simulink model "Lab8a"  (Simulink 7.4)
settings: Solver=ode23tb  StartTime=0.0  StopTime=0.2  MaxStep=100e-6  RelTol=1e-3
libraries: powerlib x5, powerlib_extras x2
settings Model: Creator=msse9  LastModifiedBy=msse9

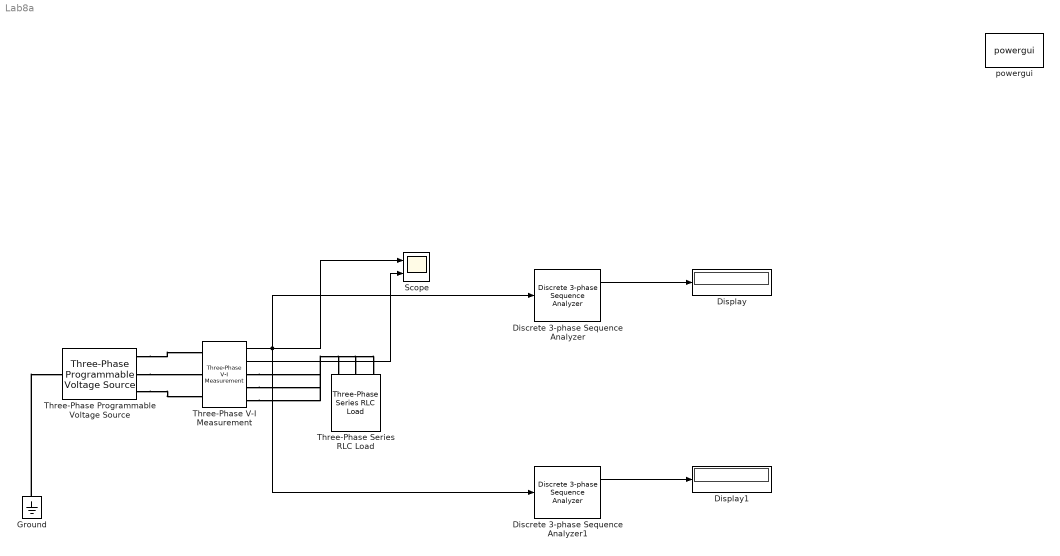
== system Lab8a ==
  Discrete 3-phase Sequence Analyzer : powerlib_extras/Discrete Measurements/Discrete 3-phase Sequence Analyzer  DialogController=POWERSYS.PowerSysDialog  SystemSampleTime=-1  Freq=50  n=3  seq=Zero  Par_Init=[0 0]  Ts=50e-6
  Discrete 3-phase Sequence Analyzer1 : powerlib_extras/Discrete Measurements/Discrete 3-phase Sequence Analyzer  DialogController=POWERSYS.PowerSysDialog  SystemSampleTime=-1  Freq=50  n=1  seq=Positive  Par_Init=[0 0]  Ts=50e-6
  Display : Display
  Display1 : Display
  Ground : powerlib/Elements/Ground  DialogController=POWERSYS.PowerSysDialog  PhysicalDomain=powersysdomain  SubClassName=unknown  LeftPortType=p1  RightPortType=p1  LConnTagsString=a
  Scope : Scope  NumInputPorts=2
      settings: YMin=-5~-5  YMax=5~5  SaveName=Lab8  SampleInput=on  SampleTime=100e-6
  Three-Phase Programmable Voltage Source : powerlib/Electrical Sources/Three-Phase Programmable Voltage Source  DialogController=POWERSYS.PowerSysDialog  SystemSampleTime=-1  PositiveSequence="[400  0 50]"  VariationEntity=None  VariationType=Step  VariationStep=0.5  VariationRate=10  VariationMagnitude=0.3  VariationFrequency=2  VariationTiming=[1 2]  VariationPhaseA=off  Amplitudes=[1 0.8 1.2 1.0]  TimeValues=[0 0.1 0.15 0.2]  HarmonicGeneration=on  HarmonicA=[3 0.2 0 0]  HarmonicB=[5 0.3 0 2]  Timing="[0.1  1]"
  Three-Phase Series RLC Load : powerlib/Elements/Three-Phase Series RLC Load  DialogController=POWERSYS.PowerSysDialog  PhysicalDomain=powersysdomain  SubClassName=unknown  LeftPortType=p1  RightPortType=p1  LConnTagsString=A|B|C  Configuration=Y (grounded)  NominalVoltage=400  NominalFrequency=50  ActivePower=1000  InductivePower=1000  CapacitivePower=0  Measurements=None
  Three-Phase V-I Measurement : powerlib/Measurements/Three-Phase V-I Measurement  DialogController=POWERSYS.PowerSysDialog  SystemSampleTime=-1  VoltageMeasurement=phase-to-ground  SetLabelV=off  LabelV=Vabc  Vpu=off  CurrentMeasurement=yes  SetLabelI=off  LabelI=Iabc  Ipu=off  Pbase=100e6  Vbase=500e3  OutputType=Complex  PhasorSimulation=off  PSBequivalent=0
  powergui : powerlib/powergui  Priority=1  SystemSampleTime=-1  SimulationMode=Continuous  SampleTime=50e-6  frequency=60  SPID=off  DisableSnubberDevices=off  DisableRonSwitches=off  DisableVfSwitches=off  SwTol=0  Interpol=off  frequencyindice=50  echomessages=off  HookPort=off  DisplayEquations=off  FunctionMessages=off  EnableUseOfTLC=off  x0status=blocks  RestoreLinks=warning  Frange=[0:2:500]  Ylog=off  Xlog=on  ShowGrid=off  save=off  variable=ZData  structure=Lab8  ZoomFFT=off  StartTime=0.15  cycles=2  DisplayStyle=1  fundamental=50  FreqAxis=on  MaxFrequency=1000  frequencyindicesteady=1  RmsSteady=1  display=off  Ts=0  methode=off
  wires:
  Three-Phase V-I Measurement/1 -> Scope/1, Discrete 3-phase Sequence Analyzer/1, Discrete 3-phase Sequence Analyzer1/1
  Three-Phase V-I Measurement/2 -> Scope/2
  Discrete 3-phase Sequence Analyzer/1 -> Display/1
  Discrete 3-phase Sequence Analyzer1/1 -> Display1/1
  connections:
  Ground/LConn1 -- Three-Phase Programmable Voltage Source/LConn1
  Three-Phase Programmable Voltage Source/RConn2 -- Three-Phase V-I Measurement/LConn2
  Three-Phase Programmable Voltage Source/RConn1 -- Three-Phase V-I Measurement/LConn1
  Three-Phase Programmable Voltage Source/RConn3 -- Three-Phase V-I Measurement/LConn3
  Three-Phase V-I Measurement/RConn1 -- Three-Phase Series RLC Load/LConn1
  Three-Phase V-I Measurement/RConn2 -- Three-Phase Series RLC Load/LConn2
  Three-Phase V-I Measurement/RConn3 -- Three-Phase Series RLC Load/LConn3
